simulink subsystem "StudentTemplate_M2a"  (R2025a)
settings: Solver=VariableStepAuto  StartTime=0.0  StopTime=10.0  RelTol=1e-3
libraries: eeGeneralControl x3, slpidlib x1
settings Model: Creator=JesseJabezArendse  LastModifiedBy=llamalulu

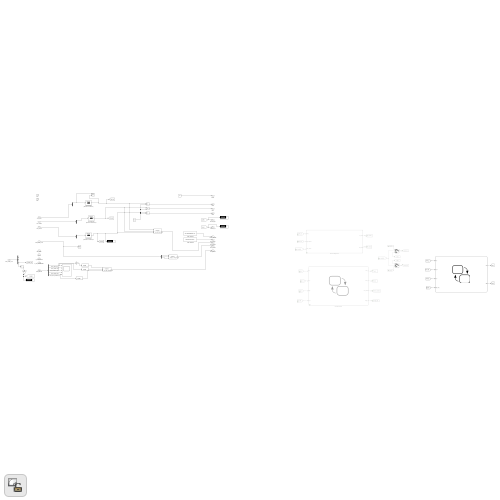
[thumbnail: Simulink's stored preview of the top-level diagram]
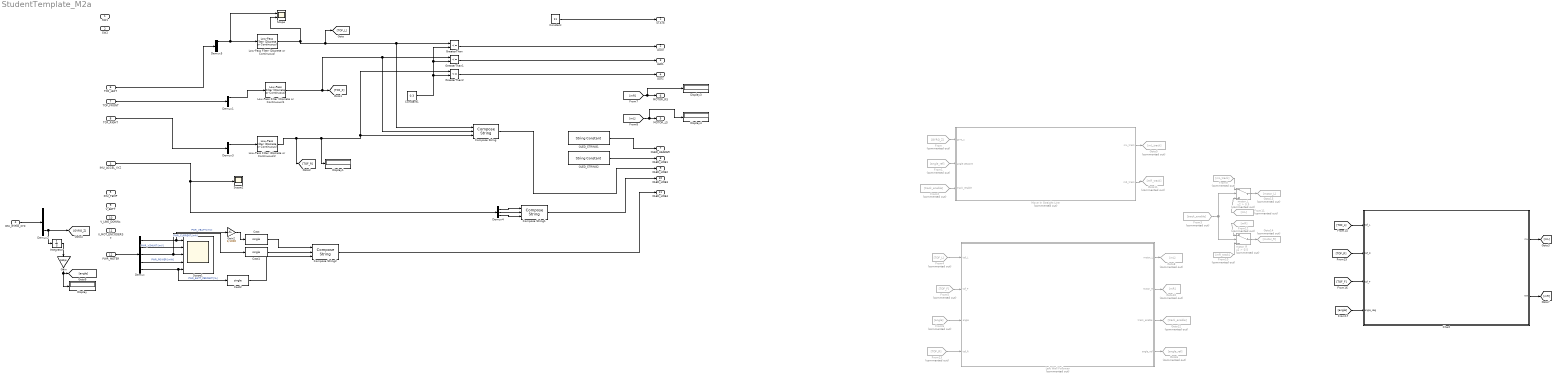
== system StudentTemplate_M2a ==
  SW1 : Inport
  SW2 : Inport  Port=2
  IMU_ACCEL_XYZ : Inport  Port=3
  IMU_GYRO_XYZ : Inport  Port=4
  IMU_TEMP : Inport  Port=5
  TOF_LEFT : Inport  Port=6
  TOF_FRONT : Inport  Port=7
  TOF_RIGHT : Inport  Port=8
  V_BATT : Inport  Port=9
  V_LINE_DOWNs : Inport  Port=10
  V_MOT_ENCODERSs : Inport  Port=11
  PWR_METER : Inport  Port=12
  Cast : DataTypeConversion  OutDataTypeStr=single  SaturateOnIntegerOverflow=off  RndMeth=Floor
  Cast1 : DataTypeConversion  OutDataTypeStr=single  SaturateOnIntegerOverflow=off  RndMeth=Floor
  Cast2 : DataTypeConversion  OutDataTypeStr=single  SaturateOnIntegerOverflow=off  RndMeth=Floor
  Chart : Stateflow chart  TreatAsAtomicUnit=on
  Compose String : ComposeString  Format="\"L%1.2f F%1.2f R%1.2f\""
  Compose String1 : ComposeString  Format="\"X%2.1f  Y%2.1f  Z%2.1f\""
  Compose String2 : ComposeString  Format="\"%1.2fV  %3.0fmA  %2.0f%%\""
  Constant : Constant  Value=11
  Constant1 : Constant  Value=0.3  SampleTime=-1
  Demux : Demux  Outputs=5
  Demux1 : Demux
  Demux2 : Demux  Outputs=3
  Demux3 : Demux
  Demux4 : Demux  Outputs=3
  Demux5 : Demux
  Display{,1,3..4} (4 alike) : Display
  From : From  Commented=on  GotoTag=GYRO_Z
  From1 : From  Commented=on  GotoTag=angle_ref
  From10 : From  Commented=on  GotoTag=mR_track
  From11 : From  Commented=on  GotoTag=mL
  From12 : From  Commented=on  GotoTag=mR
  From13 : From  Commented=on  GotoTag=TOF_R
  From2 : From  Commented=on  GotoTag=track_enable
  From3 : From  Commented=on  GotoTag=track_enable
  From4 : From  Commented=on  GotoTag=TOF_L
  From5 : From  Commented=on  GotoTag=TOF_F
  From6 : From  Commented=on  GotoTag=angle
  From9 : From  Commented=on  GotoTag=mL_track
  Gain : Gain  Gain=180/pi
  Gain2 : Gain  Gain=1/1000
  Goto10 : Goto  Commented=on  GotoTag=mR
  Goto11 : Goto  Commented=on  GotoTag=mR_track
  Goto12 : Goto  Commented=on  GotoTag=track_enable
  Goto13 : Goto  Commented=on  GotoTag=motor_L
  Goto14 : Goto  Commented=on  GotoTag=motor_R
  Goto5 : Goto  Commented=on  GotoTag=mL_track
  Goto6 : Goto  Commented=on  GotoTag=angle_ref
  Goto8 : Goto  Commented=on  GotoTag=mL
  GreaterThan : RelationalOperator  Operator=<=  OutDataTypeStr=boolean  RndMeth=Simplest  InputSameDT=off
  GreaterThan1 : RelationalOperator  Operator=<=  OutDataTypeStr=boolean  RndMeth=Simplest  InputSameDT=off
  GreaterThan2 : RelationalOperator  Operator=<=  OutDataTypeStr=boolean  RndMeth=Simplest  InputSameDT=off
  Integrator : Integrator
  Left Wall Follower : Stateflow chart  Commented=on  TreatAsAtomicUnit=on
  Low-Pass Filter (Discrete or Continuous) : eeGeneralControl/Low-Pass Filter (Discrete or Continuous)  K=1  T=0.1  B=inf  A=-inf  init_option=Inherited from block input  x0=0  Ts=-1
  Low-Pass Filter (Discrete or Continuous)1 : eeGeneralControl/Low-Pass Filter (Discrete or Continuous)  K=1  T=0.1  B=inf  A=-inf  init_option=Inherited from block input  x0=0  Ts=-1
  Low-Pass Filter (Discrete or Continuous)2 : eeGeneralControl/Low-Pass Filter (Discrete or Continuous)  K=1  T=0.1  B=inf  A=-inf  init_option=Inherited from block input  x0=0  Ts=-1
  Move In Straight Line : Subsystem  Commented=on
  OLED_STRING1 : StringConstant  String="\"UCT MICROMOUSE '25\""
  OLED_STRING2 : StringConstant  String="\"Simulink Data Demo\""
  Scope : Scope  NumInputPorts=2
      settings: ActiveDisplayYMinimum=0.22759  ActiveDisplayYMaximum=0.52326
  Scope1 : Scope  NumInputPorts=5
      settings: ActiveDisplayYMinimum=-437.5  ActiveDisplayYMaximum=3937.5  DataLoggingVariableName=ScopeData2
  Scope2 : Scope
  motor_L : Switch  Commented=on  Criteria=u2 > Threshold  Threshold=0.5  SaturateOnIntegerOverflow=off  InputSameDT=off
  motor_R : Switch  Commented=on  Criteria=u2 > Threshold  Threshold=0.5  SaturateOnIntegerOverflow=off  InputSameDT=off
  STATE : Outport
  LED0 : Outport  Port=2
  LED1 : Outport  Port=3
  LED2 : Outport  Port=4
  MOTOR_LS : Outport  Port=5
  MOTOR_RS : Outport  Port=6
  OLED_HEADER : Outport  Port=7
  OLED_LINE1 : Outport  Port=8
  OLED_LINE2 : Outport  Port=9
  OLED_LINE3 : Outport  Port=10
  OLED_LINE4 : Outport  Port=11
  wires:
  OLED_STRING2/1 -> OLED_LINE1/1
  Compose String1/1 -> OLED_LINE3/1
  Low-Pass Filter (Discrete or Continuous)1/1 -> Compose String/2, GreaterThan1/1, [TOF_F]
  GreaterThan1/1 -> LED1/1
  OLED_STRING1/1 -> OLED_HEADER/1
  TOF_LEFT/1 -> Demux5/1
  Compose String/1 -> OLED_LINE2/1
  Constant1/1 -> GreaterThan2/2, GreaterThan1/2, GreaterThan/2
  GreaterThan2/1 -> LED2/1
  GreaterThan/1 -> LED0/1
  PWR_METER/1 -> Demux/1
  Demux/1 -> Scope1/1, Gain2/1  "PWR_VBATT [mV]"
  Demux/2 -> Scope1/2  "PWR_VSHUNT [mV]"
  Demux/3 -> Scope1/3, Cast1/1  "PWR_CURRENT [mA]"
  Demux/4 -> Scope1/4  "PWR_POWER [mW]"
  Demux/5 -> Scope1/5, Cast2/1  "PWR_BATT_PERCENT [%]"
  IMU_ACCEL_XYZ/1 -> Demux4/1, Scope2/1
  Demux4/1 -> Compose String1/1
  Demux4/2 -> Compose String1/2
  Demux4/3 -> Compose String1/3
  Compose String2/1 -> OLED_LINE4/1
  Gain2/1 -> Cast/1
  Cast/1 -> Compose String2/1
  Cast1/1 -> Compose String2/2
  Cast2/1 -> Compose String2/3
  Low-Pass Filter (Discrete or Continuous)2/1 -> Compose String/3, GreaterThan2/1, Display1/1, [TOF_R]
  Low-Pass Filter (Discrete or Continuous)/1 -> Scope/2, Compose String/1, GreaterThan/1, [TOF_L]
  Constant/1 -> STATE/1
  TOF_FRONT/1 -> Demux1/1
  Demux1/1 -> Low-Pass Filter (Discrete or Continuous)1/1
  Demux3/1 -> Low-Pass Filter (Discrete or Continuous)2/1
  TOF_RIGHT/1 -> Demux3/1
  Demux5/1 -> Low-Pass Filter (Discrete or Continuous)/1, Scope/1
  IMU_GYRO_XYZ/1 -> Demux2/1
  Demux2/3 -> [GYRO_Z], Integrator/1
  Move In Straight Line/1(mL_track) -> Goto5/1
  Integrator/1 -> Gain/1
  Gain/1 -> Display/1, [angle]
  From4/1 -> Left Wall Follower/1(tof_L)
  From5/1 -> Left Wall Follower/2(tof_F)
  From6/1 -> Left Wall Follower/3(angle)
  Left Wall Follower/1(motor_L) -> Goto8/1
  Left Wall Follower/2(motor_R) -> Goto10/1
  Move In Straight Line/2(mR_track) -> Goto11/1
  From3/1 -> motor_R/2, motor_L/2
  From11/1 -> motor_L/3
  From12/1 -> motor_R/1
  From10/1 -> motor_R/3
  From9/1 -> motor_L/1
  motor_L/1 -> Goto13/1
  motor_R/1 -> Goto14/1
  From/1 -> Move In Straight Line/1(gyro_z)
  Left Wall Follower/4(angle_ref) -> Goto6/1
  From1/1 -> Move In Straight Line/2(angle setpoint)
  From2/1 -> Move In Straight Line/3(track_enable)
  Left Wall Follower/3(track_enable) -> Goto12/1
  [mR] -> MOTOR_RS/1, Display3/1
  [mL] -> MOTOR_LS/1, Display4/1
  From13/1 -> Left Wall Follower/4(tof_R)
  [TOF_L] -> Chart/1(tof_L)
  [TOF_R] -> Chart/2(tof_R)
  [TOF_F] -> Chart/3(tof_F)
  [angle] -> Chart/4(angle_deg)
  Chart/1(mL) -> [mL]
  Chart/2(mR) -> [mR]

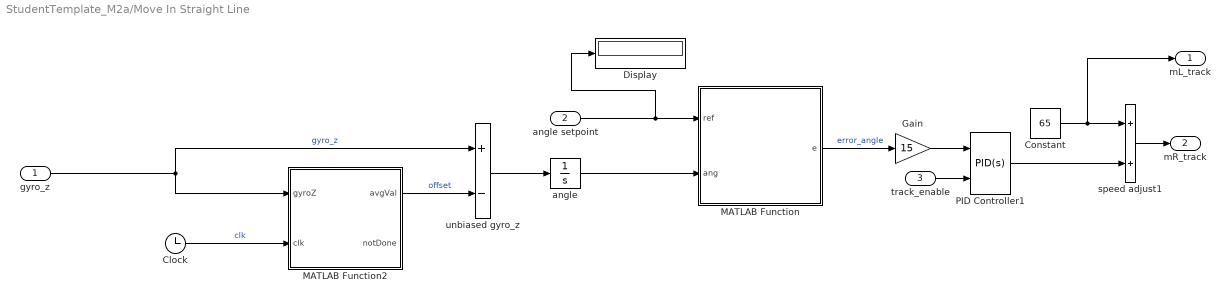
== system StudentTemplate_M2a/Move In Straight Line ==
  gyro_z : Inport
  angle setpoint : Inport  Port=2
  track_enable : Inport  Port=3
  Clock : Clock
  Constant : Constant  Value=65
  Display : Display
  Gain : Gain  Gain=15
  MATLAB Function : MATLAB Function  TreatAsAtomicUnit=on
  MATLAB Function2 : MATLAB Function  TreatAsAtomicUnit=on  SystemSampleTime=0.01
  PID Controller1 : slpidlib/PID Controller  Controller=PID  Form=Parallel  TimeDomain=Continuous-time  UseExternalTs=off  SampleTime=-1  IntegratorMethod=Forward Euler  FilterMethod=Forward Euler  ControllerParametersSource=internal  P=1  I=1  UseKiTs=off  D=0  UseExternalDerivativeSource=off  N=100  UseFilter=on  TunerSelectOption=Transfer Function Based (PID Tuner App)  InitialConditionSource=internal  InitialConditionForIntegrator=0  InitialConditionForFilter=0  DifferentiatorICPrevScaledInput=0  ExternalReset=rising  TrackingMode=off  Kt=1  LimitOutput=off  SatLimitsSource=internal  UpperSaturationLimit=inf  LowerSaturationLimit=-inf  LinearizeAsGain=on  AntiWindupMode=none  Kb=1  LimitIntegrator=off  UpperIntegratorSaturationLimit=inf  LowerIntegratorSaturationLimit=-inf  RndMeth=Round  POutMin=[]  POutMax=[]  IOutMin=[]  IOutMax=[]  DOutMin=[]  DOutMax=[]  NOutMin=[]  NOutMax=[]  SumOutMin=[]  SumOutMax=[]  SaturationOutMin=[]  SaturationOutMax=[]  PParamMin=[]  PParamMax=[]  IParamMin=[]  IParamMax=[]  DParamMin=[]  DParamMax=[]  NParamMin=[]  NParamMax=[]  KbParamMin=[]  KbParamMax=[]  KtParamMin=[]  KtParamMax=[]  KbOutMin=[]  KbOutMax=[]  KtOutMin=[]  KtOutMax=[]  IntegratorOutMin=[]  IntegratorOutMax=[]  FilterOutMin=[]  FilterOutMax=[]  SumI1OutMin=[]  SumI1OutMax=[]  SumI2OutMin=[]  SumI2OutMax=[]  SumI3OutMin=[]  SumI3OutMax=[]  SumI4OutMin=[]  SumI4OutMax=[]  SumDOutMin=[]  SumDOutMax=[]  DifferentiatorOutMin=[]  DifferentiatorOutMax=[]  FilterDiffOutCoefMin=[]  FilterDiffOutCoefMax=[]  ReciprocalOutMin=[]  ReciprocalOutMax=[]  SumDenOutMin=[]  SumDenOutMax=[]  SumNumOutMin=[]  SumNumOutMax=[]  DivideOutMin=[]  DivideOutMax=[]  UdiffTsProdOutMin=[]  UdiffTsProdOutMax=[]  NTsProdOutMin=[]  NTsProdOutMax=[]  UintegralTsProdOutMin=[]  UintegralTsProdOutMax=[]  UngainTsProdOutMin=[]  UngainTsProdOutMax=[]  ClampingZeroOutDataTypeStr=Inherit: Inherit via back propagation  ClampingZeroOutMin=[]  ClampingZeroOutMax=[]  FilterDenConstantOutDataTypeStr=Inherit: Inherit via back propagation  FilterDenConstantOutMin=[]  FilterDenConstantOutMax=[]  PCopyOutDataTypeStr=Inherit: Inherit via back propagation  PCopyOutMin=[]  PCopyOutMax=[]  NCopyOutDataTypeStr=Inherit: Inherit via back propagation  NCopyOutMin=[]  NCopyOutMax=[]  IntegratorContinuousStateAttributes=''  IntegratorStateMustResolveToSignalObject=off  IntegratorRTWStateStorageClass=Auto  FilterContinuousStateAttributes=''  FilterStateMustResolveToSignalObject=off  FilterRTWStateStorageClass=Auto  ParallelPVariant=InternalParameters  IdealPVariant=Disabled  IVariant=InternalParameters  DVariant=InternalParameters  IntegratorVariant=Continuous  SatVariant=Disabled  AWVariant=Passthrough  PCopyVariant=Disabled  TRVariant=Disabled  FdbkBlocksVariant=Forward  IdealPFdbkVariant=Disabled  SatFdbkVariant=Disabled  DerivativeFilterVariant=ContFilter  NVariant=InternalParameters  NCopyVariant=Disabled  FilterICVariant=InternalICsFilter  IntegratorICVariant=InternalICs  ExternalResetVariant=ExternalReset  TRSumVariant=Passthrough  SumFdbkVariant=Disabled  SumVariant=Sum_PID  TsampFilterVariant=InternalTs  TsampNgainVariant=Passthrough  TsampIntegralVariant=Disabled_SignalSpec  ExternalSaturationOutDataTypeStr=Inherit: Same as second input  DerivativeSourceVariant=ErrorSignal  PreIntVariant=InternalPreInt
  angle : Integrator
  speed adjust1 : Sum
  unbiased gyro_z : Sum  Inputs=+-
  mL_track : Outport
  mR_track : Outport  Port=2
  wires:
  track_enable/1 -> PID Controller1/2
  angle setpoint/1 -> MATLAB Function/1(ref), Display/1
  angle/1 -> MATLAB Function/2(ang)
  Constant/1 -> speed adjust1/1, mL_track/1
  speed adjust1/1 -> mR_track/1
  unbiased gyro_z/1 -> angle/1
  PID Controller1/1 -> speed adjust1/2
  Gain/1 -> PID Controller1/1
  gyro_z/1 -> MATLAB Function2/1(gyroZ), unbiased gyro_z/1  "gyro_z"
  Clock/1 -> MATLAB Function2/2(clk)  "clk"
  MATLAB Function2/1(avgVal) -> unbiased gyro_z/2  "offset"
  MATLAB Function/1(e) -> Gain/1  "error_angle"

== stateflow chart StudentTemplate_M2a/Chart ==
  state MoveForward
    entry:
    mL = BASE_SPEED;
    mR = BASE_SPEED;
    update_flags();
    during:
    update_flags();
  state AfterTurn
    entry:
    mL = BASE_SPEED;
    mR = BASE_SPEED;
    start_dist = tof_F;
    dist_travelled = 0;
    update_flags();
    during:
    dist_travelled = start_dist - tof_F;
    update_flags();
  state LeftJunc
    entry:
    mL = BASE_SPEED; mR = BASE_SPEED;
    start_dist = tof_F; dist_travelled = 0;
    update_flags();
    during:
    dist_travelled = start_dist - tof_F;
    update_flags();
  state TurnLeft
    entry:
    target_angle = target_angle + 90;     % +90° from last target
    mL = -TURN_SPEED;
    mR =  TURN_SPEED;
  state TurnRight
    entry:
    target_angle = target_angle - 90;    % -90°
    mL =  TURN_SPEED;
    mR = -TURN_SPEED;
  (default) -> MoveForward : { target_angle = angle_deg; mL = 0; mR = 0; update_flags(); }
  AfterTurn -> MoveForward [order 2] : [(dist_travelled > NXT_BLOCK) && (LEFT_OPEN || RIGHT_OPEN || FRONT_BLOCKED)]
  MoveForward -> LeftJunc [order 2] : [LEFT_OPEN]
  MoveForward -> (junction 75) [order 1] : [FRONT_BLOCKED]
  AfterTurn -> (junction 75) [order 1] : [FRONT_BLOCKED]
  LeftJunc -> (junction 75) : [dist_travelled > BLOCK_ADV || FRONT_BLOCKED]
  (junction 75) -> TurnLeft [order 1] : [LEFT_OPEN || (LEFT_BLOCKED && RIGHT_BLOCKED)]
  (junction 75) -> TurnRight [order 2] : [RIGHT_OPEN]
  (junction 82) -> AfterTurn
  AfterTurn -> TurnLeft [order 3] : [LEFT_OPEN && (dist_travelled > NXT_BLOCK)]
  TurnLeft -> (junction 82) : [angle_deg >= target_angle]
  TurnRight -> (junction 82) : [angle_deg <= target_angle]
  data: tof_L input; tof_R input; tof_F input; angle_deg input; mL output double; mR output double; BASE_SPEED constant double =60; TURN_SPEED constant double =25; L_detect constant double =0.15; R_detect constant double =0.15; target_angle local; start_dist local; dist_travelled local; BLOCK_ADV constant double =0.135; NXT_BLOCK constant double =0.2; F_detect constant double =0.05; LEFT_OPEN local boolean; LEFT_BLOCKED local boolean; RIGHT_OPEN local boolean; RIGHT_BLOCKED local boolean; FRONT_BLOCKED local boolean
  function update_flags:
    | function update_flags()
    | LEFT_OPEN     = (tof_L >  L_detect);
    | LEFT_BLOCKED  = (tof_L <= L_detect);
    | 
    | RIGHT_OPEN    = (tof_R >  R_detect);
    | RIGHT_BLOCKED = (tof_R <= R_detect);
    | 
    | FRONT_BLOCKED = (tof_F <= F_detect);

== stateflow chart StudentTemplate_M2a/Left Wall Follower ==
  state UTurn
    entry:
    angle_ref   = angle;
    turn_target = uturn180(angle_ref);
    motor_L = -v_turn;
    motor_R = v_turn;
    during:
    if abs(ang_err(angle, turn_target)) <= angle_tol
    motor_L = 0;
    motor_R = 0;
    end
  state Track
    during:
    motor_L = 65;
    motor_R = 65;
  state SeekWall
    during:
    motor_L = -v_turn;   % turn in place left
    motor_R =  v_turn;
  state DeadEnd
    entry:
    motor_L = 0;
    motor_R = 0;
  state Boot
    entry:
    motor_L = 0;
    motor_R = 0;
    angle_ref = angle;
    track_enable = 0;
  state TurnLeft
    entry:
    angle_ref   = angle;
    turn_target = left90(angle_ref);
    motor_L = -v_turn;
    motor_R =  v_turn;
    during:
    if abs(ang_err(angle, turn_target)) <= angle_tol
    motor_L = 0;
    motor_R = 0;
    end
  state TurnRight
    entry:
    angle_ref   = angle;
    turn_target = right90(angle_ref);
    motor_L = v_turn;
    motor_R = -v_turn;
    during:
    if abs(ang_err(angle, turn_target)) <= angle_tol
    motor_L = 0;
    motor_R = 0;
    end
  DeadEnd -> UTurn
  UTurn -> SeekWall : [ abs(ang_err(angle, turn_target)) <= angle_tol ]
  (junction 68) -> SeekWall
  SeekWall -> Track : [ LEFT_WALL && FRONT_CLEAR ]
  Boot -> SeekWall [order 1] : [tof_L > L_detect]
  (default) -> Boot
  Track -> DeadEnd [order 1] : [ FRONT_BLOCK && LEFT_WALL && RIGHT_WALL ]
  Boot -> Track [order 2] : [ tof_L <= L_detect && tof_F > F_clear ]
  Track -> TurnLeft [order 2] : [ LEFT_OPEN ]
  TurnLeft -> Track [order 1] : [ abs(ang_err(angle, turn_target)) <= angle_tol ]
  Track -> TurnRight [order 3] : [ FRONT_BLOCK && LEFT_WALL && RIGHT_OPEN ]
  TurnRight -> Track [order 1] : [ abs(ang_err(angle, turn_target)) <= angle_tol ]
  TurnLeft -> (junction 68) [order 2] : [ abs(ang_err(angle, turn_target)) <= angle_tol && (tof_F <= F_clear) ]
  TurnRight -> (junction 68) [order 2] : [ abs(ang_err(angle, turn_target)) <= angle_tol && (tof_F <= F_clear) ]
  data: curr_deg function_input; target_deg function_input; e function_output; a function_input; a function_output; curr_ref function_input; t function_output; curr_ref function_input; t function_output; curr_ref function_input; t function_output; tof_L input; tof_F input; angle input; motor_L output; motor_R output; L_detect constant double =0.16; L_corner constant double =0.06; L_open constant double =0.3; v_turn constant double =55; turn_target local; angle_tol constant double =1; F_clear constant double =0.13; track_enable output; angle_ref output; FRONT_CLEAR local boolean =tof_F > F_clear; FRONT_BLOCK local boolean =tof_F <= F_clear; LEFT_WALL local boolean =tof_L <= L_detect; LEFT_OPEN local boolean =tof_L >= L_open; RIGHT_WALL local boolean =tof_R <= R_detect; RIGHT_OPEN local boolean =tof_R >= R_open; tof_R input
  function e = ang_err(curr_deg, target_deg):
    | function e = ang_err(curr_deg, target_deg)
    | % Returns signed shortest error in degrees in [-180, +180]
    | e = target_deg - curr_deg;
    | e = mod(e + 180, 360) - 180;
  function a = wrap360(a):
    | function a = wrap360(a)
    | a = mod(a, 360);
    | if a < 0
    |     a = a + 360;
    | end
  function t = left90(curr_ref):
    | function t = left90(curr_ref)
    | t = wrap360(curr_ref + 90);
  function t = right90(curr_ref):
    | function t = right90(curr_ref)
    | t = wrap360(curr_ref - 90);
  function t = uturn180(curr_ref):
    | function t = uturn180(curr_ref)
    | t = wrap360(curr_ref + 180);

== matlab function StudentTemplate_M2a/Move In Straight Line/MATLAB Function ==
  data: ref input; e output; ang input
function e = wrapErrDeg(ref, ang)
e = ref - ang;
e = mod(e + 180, 360) - 180;   % -> (-180,180]

== matlab function StudentTemplate_M2a/Move In Straight Line/MATLAB Function2 ==
  data: gyroZ input; avgVal output; notDone output; clk input
function [avgVal, notDone] = avgGyroZ(gyroZ, clk)
% avgGyroZ - Calculates the average of the first 1000 gyro z-axis readings.
% Once 1000 samples are collected, it locks the average and sets 'done' to true.
%
% Inputs:
%   gyroZ - new single gyro z-axis reading (scalar)
%
% Outputs:
%   avgVal - constant average of the first 100 samples once done = true
%   done   - boolean flag, true when average has been calculated

    % Persistent variables to store data between calls
    persistent buffer count lockedAvg
    notDone = true;
    avgVal = 0;
    length = 1000;
    
    % Initialise on first run
    if isempty(buffer)
        buffer = zeros(1,length); 
        count = 0;
        lockedAvg = 0; % Not ready yet
    end
    
    if clk > 0.5
	    % Increment sample count and store new reading (until 100 readings reached)
	    if count < length
	        count = count + 1;
	        buffer(count) = gyroZ;
	        
	        notDone = true;
	        avgVal = 0;
	        
	        % When we hit 100 samples, calculate and lock average
	        if count == length
	            lockedAvg = mean(buffer);
	            notDone = false;
	            avgVal = lockedAvg;
	        end
	    else
	        % Already locked: always output the same average
	        notDone = false;
	        avgVal = lockedAvg;
	    end
	 end
end
